simulink subsystem "Velocity_Profiles"  (R2023a)
settings: Solver=VariableStepAuto  StartTime=0.0  StopTime=10.0  RelTol=1e-3

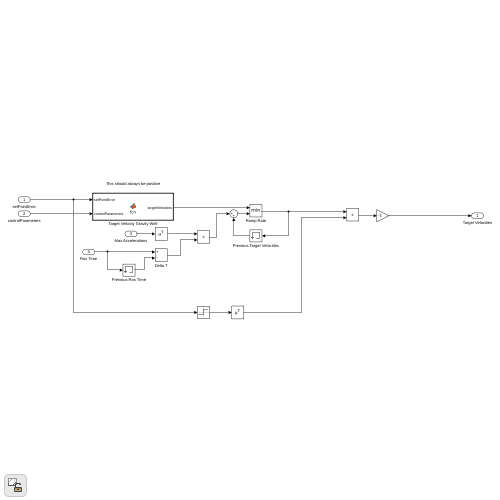
[thumbnail: Simulink's stored preview of the top-level diagram]
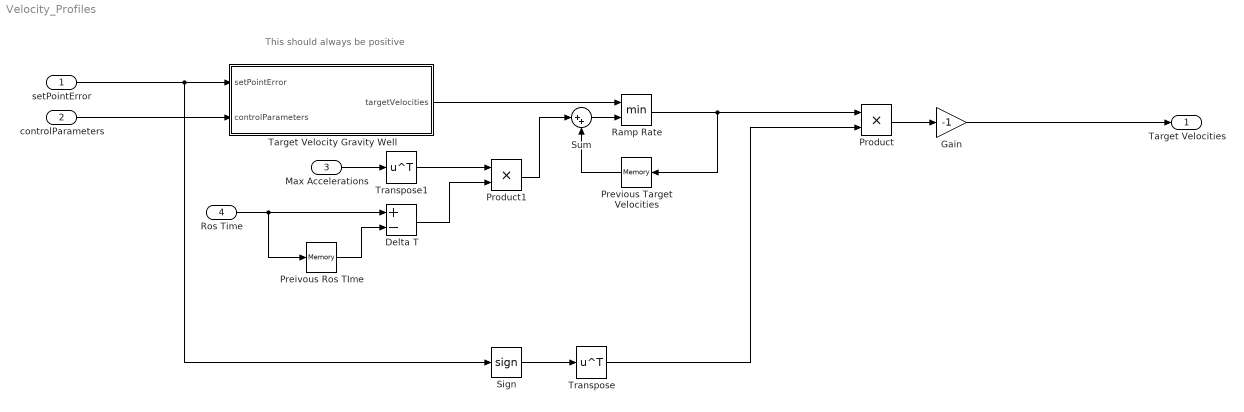
== system Velocity_Profiles ==
  note: This should always be positive
  setPointError : Inport
  controlParameters : Inport  Port=2
  Max Accelerations : Inport  Port=3
  Ros Time : Inport  Port=4
  Delta T : Sum  Inputs=+-
  Gain : Gain  Gain=-1
  Preivous Ros TIme : Memory
  Previous Target Velocities : Memory
  Product : Product
  Product1 : Product
  Ramp Rate : MinMax  Inputs=2
  Sign : Signum
  Sum : Sum  Inputs=|++
  Target Velocity Gravity Well : MATLAB Function  TreatAsAtomicUnit=on
  Transpose : Math  Operator=transpose
  Transpose1 : Math  Operator=transpose
  Target Velocities : Outport
  wires:
  Transpose1/1 -> Product1/1
  Max Accelerations/1 -> Transpose1/1
  Transpose/1 -> Product/2
  controlParameters/1 -> Target Velocity Gravity Well/2(controlParameters)
  Ramp Rate/1 -> Product/1, Previous Target Velocities/1
  Gain/1 -> Target Velocities/1
  Product1/1 -> Sum/1
  Preivous Ros TIme/1 -> Delta T/2
  Previous Target Velocities/1 -> Sum/2
  Sign/1 -> Transpose/1
  Ros Time/1 -> Delta T/1, Preivous Ros TIme/1
  Product/1 -> Gain/1
  Target Velocity Gravity Well/1(targetVelocities) -> Ramp Rate/1
  Delta T/1 -> Product1/2
  Sum/1 -> Ramp Rate/2
  setPointError/1 -> Sign/1, Target Velocity Gravity Well/1(setPointError)

== matlab function Velocity_Profiles/Target Velocity Gravity Well ==
function targetVelocities = fcn(setPointError, controlParameters)

%the target velocities to converge to - this should always be positive
targetVelocities = zeros(6,1);

controlParametersExpectedLength = 12;
if(~length(controlParameters) == controlParametersExpectedLength)
    %params have not yet been assigned / assgined incorrectly
    return
end

controlParameters = reshape(controlParameters, [length(controlParameters) / 6, 6]);
%param(1,x) = max control value
%param(2,x) = the error where max control is reached

%velocity curves = param(1,x) * (-cos(error * pi / (2 * param(2,x)))^1/2 + 1)
for i=1:6
    if(controlParameters(2, i) == 0 || setPointError(i) == 0)
        targetVelocities(i) = 0;
    else
        %ensure the saturation error is not exceeded
        if(abs(setPointError(i)) > controlParameters(2, i))
            setPointError(i) = controlParameters(2, i) * setPointError(i) / abs(setPointError(i));
        end

        targetVelocities(i) = controlParameters(1,i) * (-abs(cos(setPointError(i) * pi / (2 * controlParameters(2,i))))^(1/2) + 1);
    end


end
